simulink model "resonance_step"  (R2022a)
settings: Solver=VariableStepAuto  StartTime=0.0  StopTime=27  MaxStep=1e-3  RelTol=1e-3
undefined symbols (not defined in the file): i
libraries: resonance_lib x1
settings Model: Creator=tstef  LastModifiedBy=thomas

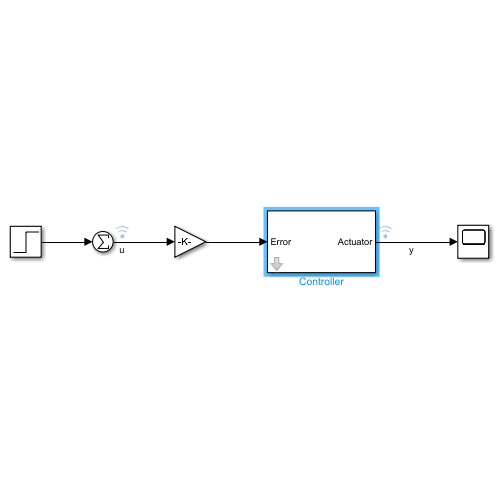
[thumbnail: Simulink's stored preview of the top-level diagram]
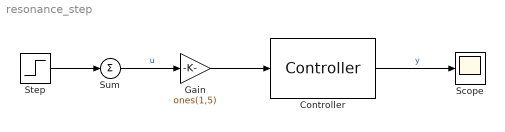
== system resonance_step ==
  Controller : resonance_lib/Controller  k_P=43  k_I=10  k_R=95-390*i  k_Ra=950  k_Rb=-3.9e5  k_PIRA=4.1e5  k_PIRAp=-210  k_PIRAz=21  T1=0.094  T1p=-210  T1z=21  w0=100  zeta=0.05
  Gain : Gain  Gain=ones(1,5)
  Scope : Scope
  Step : Step  Time=[0.1 9 10.3 11.2 12.57 20.57]  After=[1 -1 -1 1 -1 1]  SampleTime=0
  Sum : Sum  Inputs=+
  wires:
  Controller/1 -> Scope/1  "y"
  Gain/1 -> Controller/1
  Sum/1 -> Gain/1  "u"
  Step/1 -> Sum/1
